simulink model "V_ideal"  (Simulink 5.0)
settings: Solver=ode23tb  SolverMode=SingleTasking  StartTime=0.0  StopTime=0.1  RelTol=1e-3
libraries: powerlib2 x17, powerlib_extras x1
settings Model: Creator=sybille  LastModifiedBy=gnedin pa  ExtModeTrigMode=oneshot  ExtModeArmWhenConnect=off  SaveTime=off  SaveOutput=off  LimitDataPoints=off  UnconnectedInputMsg=none  UnconnectedOutputMsg=none  BlockReductionOpt=off  BooleanDataType=off  RTWTemplateMakefile=grt_unix.tmf

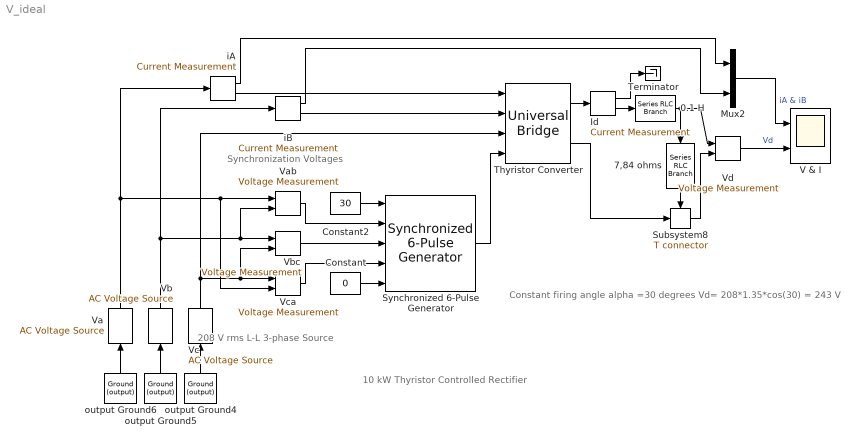
== system V_ideal ==
  note: Synchronization Voltages
  note: 208 V rms L-L
      | 3-phase Source
  note: 10 kW Thyristor Controlled Rectifier
  note: Constant firing angle alpha =30 degrees
      | Vd= 208*1.35*cos(30) = 243 V
  0.1 H : powerlib2/Elements/Series RLC Branch  Tag=PoWeRsYsTeMbLoCk  a=0  b=100e-3  c=inf  mesure=None  PSBOutputType=1
  7,84 ohms : powerlib2/Elements/Series RLC Branch  Tag=PoWeRsYsTeMbLoCk  Orientation=down  a=7.84  b=0  c=inf  mesure=None  PSBOutputType=1
  Constant : Constant  Value=0
  Constant2 : Constant  Value=30
  Id : powerlib2/Measurements/Current Measurement  Tag=PoWeRsYsTeMmEaSuReMeNt  PhasorSimulation=off  OutputType=Magnitude  PSBOutputType=01  PSBequivalent=0
  Mux2 : Mux  Inputs=2
  Subsystem8 : powerlib2/Connectors/T connector  Tag=PoWeRsYsTeMbLoCk  PSBOutputType=1
  Synchronized 6-Pulse Generator : powerlib_extras/Control  Blocks/Synchronized 6-Pulse Generator  freq=60  pwidth=10  Double_Pulse=off
  Terminator : Terminator
  Thyristor Converter : powerlib2/Power Electronics/Universal Bridge  Tag=PoWeRsYsTeMbLoCk  arms=3  confi=ABC as input terminals  injcc=500  cf=.01e-6  device=Thyristors  Ron=0.01  Lon=1e-6  VFs="[  0.8  0.8  ]"  Vf=0.8  gtoparameters=[ 10e-6 , 20e-6 ]  igbtparameters=[ 1e-6 , 2e-6 ]  mesure=Device currents  PSBOutputType=111
  V & I : Scope  NumInputPorts=2
      settings: TimeRange=0.1  YMin=-40~0  YMax=40~250  DataFormat=Structure
  Va : powerlib2/Electrical Sources/AC Voltage Source  Tag=PoWeRsYsTeMbLoCk  Orientation=up  A=208*sqrt(2/3)  P=0  F=60  stime=0  mesure=None  PSBOutputType=1
  Vab : powerlib2/Measurements/Voltage Measurement  Tag=PoWeRsYsTeMmEaSuReMeNt  PhasorSimulation=off  OutputType=Magnitude  PSBOutputType=0  PSBequivalent=0
  Vb : powerlib2/Electrical Sources/AC Voltage Source  Tag=PoWeRsYsTeMbLoCk  Orientation=up  A=208*sqrt(2/3)  P=-120  F=60  stime=0  mesure=None  PSBOutputType=1
  Vbc : powerlib2/Measurements/Voltage Measurement  Tag=PoWeRsYsTeMmEaSuReMeNt  PhasorSimulation=off  OutputType=Magnitude  PSBOutputType=0  PSBequivalent=0
  Vc : powerlib2/Electrical Sources/AC Voltage Source  Tag=PoWeRsYsTeMbLoCk  Orientation=up  A=208*sqrt(2/3)  P=120  F=60  stime=0  mesure=None  PSBOutputType=1
  Vca : powerlib2/Measurements/Voltage Measurement  Tag=PoWeRsYsTeMmEaSuReMeNt  PhasorSimulation=off  OutputType=Magnitude  PSBOutputType=0  PSBequivalent=0
  Vd : powerlib2/Measurements/Voltage Measurement  Tag=PoWeRsYsTeMmEaSuReMeNt  PhasorSimulation=off  OutputType=Magnitude  PSBOutputType=0  PSBequivalent=0
  iA : powerlib2/Measurements/Current Measurement  Tag=PoWeRsYsTeMmEaSuReMeNt  PhasorSimulation=off  OutputType=Magnitude  PSBOutputType=01  PSBequivalent=0
  iB : powerlib2/Measurements/Current Measurement  Tag=PoWeRsYsTeMmEaSuReMeNt  PhasorSimulation=off  OutputType=Magnitude  PSBOutputType=01  PSBequivalent=1
  output Ground4 : powerlib2/Connectors/Ground (output)  Tag=PoWeRsYsTeMbLoCk  Orientation=up  PSBOutputType=1
  output Ground5 : powerlib2/Connectors/Ground (output)  Tag=PoWeRsYsTeMbLoCk  Orientation=up  PSBOutputType=1
  output Ground6 : powerlib2/Connectors/Ground (output)  Tag=PoWeRsYsTeMbLoCk  Orientation=up  PSBOutputType=1
  wires:
  Thyristor Converter/1 -> Id/1
  Thyristor Converter/2 -> Subsystem8/1
  Subsystem8/1 -> Vd/2
  Vca/1 -> Synchronized 6-Pulse Generator/4
  Vbc/1 -> Synchronized 6-Pulse Generator/3
  Vab/1 -> Synchronized 6-Pulse Generator/2
  iA/2 -> Thyristor Converter/1
  iB/2 -> Thyristor Converter/2
  Constant/1 -> Synchronized 6-Pulse Generator/5
  Vc/1 -> Vca/1, Vbc/2, Thyristor Converter/3
  Vb/1 -> Vbc/1, Vab/2, iB/1
  Va/1 -> Vab/1, Vca/2, iA/1
  Synchronized 6-Pulse Generator/1 -> Thyristor Converter/4
  Constant2/1 -> Synchronized 6-Pulse Generator/1
  7,84 ohms/1 -> Subsystem8/Enable
  Id/2 -> 0.1 H/1
  0.1 H/1 -> 7,84 ohms/1, Vd/1
  iA/1 -> Mux2/1
  iB/1 -> Mux2/2
  Mux2/1 -> V & I/1  "iA & iB"
  Vd/1 -> V & I/2  "Vd"
  output Ground6/1 -> Va/1
  output Ground5/1 -> Vb/1
  output Ground4/1 -> Vc/1
  Id/1 -> Terminator/1
